simulink model "No2_WriteUORBData"  (R2022a)
settings: Solver=FixedStepAuto  StartTime=0.0  StopTime=inf  MaxStep=0.005  RelTol=1e-3  EnableMultiTasking=on
libraries: px4uORBlib x2
settings Model: ExtModeTrigDuration=10  Creator=liuwhale  LastModifiedBy=liuwhale
settings SolverCC: PositivePriorityOrder=on
settings OptimizationCC: EnhancedBackFolding=on  PassReuseOutputArgsAs=Individual arguments  ZeroExternalMemoryAtStartup=off  ZeroInternalMemoryAtStartup=off  MaxStackSize=64  OptimizeBlockOrder=speed  DifferentSizesBufferReuse=on  OptimizationCustomize=off  EfficientTunableParamExpr=on
settings DebuggingCC: ParameterTunabilityLossMsg=error
settings HardwareCC: ProdBitPerPointer=32  ProdBitPerSizeT=32  ProdBitPerPtrDiffT=32  ProdLargestAtomicInteger=Long  ProdLargestAtomicFloat=Double  ProdWordSize=32  ProdLongLongMode=on  ProdHWDeviceType=ARM Compatible->ARM Cortex
settings SFSimCC: MATLABDynamicMemAlloc=off  SimTargetLang=C++
settings RTWCC: SystemTargetFile=ert.tlc  HardwareBoard=PX4 Pixhawk 1  TLCOptions="-aInlineSetEventsForThisBaseRateFcn=TLC_FALSE -aSuppressMultiTaskScheduler=TLC_FALSE  -aRateBasedStepFcn=0"  TemplateMakefile=ert_default_tmf  Toolchain=GNU Tools for PX4 Autopilots  TargetLang=C++
settings CodeAppCC: ForceParamTrailComments=on  IgnoreCustomStorageClasses=off  OperatorAnnotations=on  SimulinkDataObjDesc=on  SFDataObjDesc=on  InsertBlockDesc=on
settings ERTTargetCC: ExtModeStaticAllocSize=1024

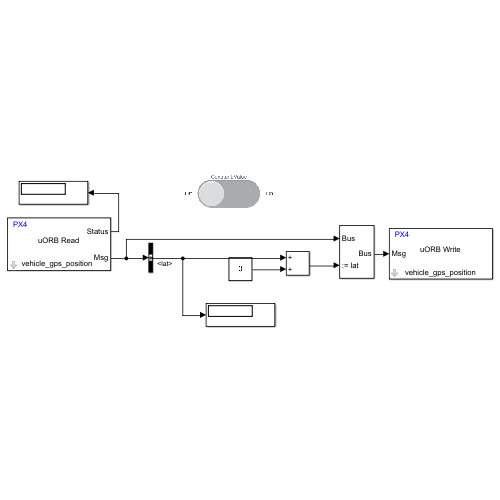
[thumbnail: Simulink's stored preview of the top-level diagram]
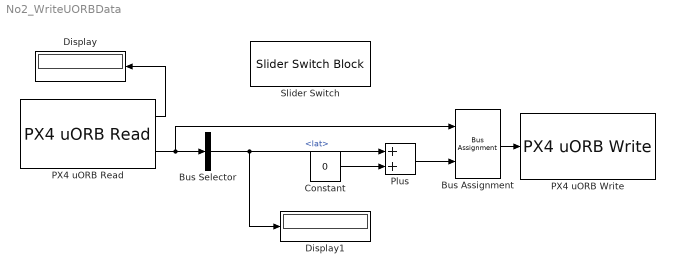
== system No2_WriteUORBData ==
  Bus Assignment : BusAssignment  AssignedSignals=lat
  Bus Selector : BusSelector  OutputSignals=lat
  Constant : Constant  Value=0
  Display : Display
  Display1 : Display
  PX4 uORB Read : px4uORBlib/PX4 uORB Read  uORBTopic=vehicle_gps_position  selectInstance=vehicle_gps_position  SampleTime=-1  BlockingMode=off  BlockTimeout=1e-3
      settings: SourceProductBaseCode=PX4AUTOPILOTS
  PX4 uORB Write : px4uORBlib/PX4 uORB Write  uORBTopic=vehicle_gps_position  selectInstance=vehicle_gps_position  MessageQueueLen=1
      settings: SourceProductBaseCode=PX4AUTOPILOTS
  Plus : Sum  OutDataTypeStr=int32
  Slider Switch : SliderSwitchBlock
      settings: Values={{'Off', 'On'}, [0 1]}
  wires:
  PX4 uORB Read/1 -> Display/1
  PX4 uORB Read/2 -> Bus Assignment/1, Bus Selector/1
  Bus Selector/1 -> Display1/1, Plus/1  "<lat>"
  Bus Assignment/1 -> PX4 uORB Write/1
  Plus/1 -> Bus Assignment/2
  Constant/1 -> Plus/2
